simulink library "turbine_ul"  (R2018b)
settings: Solver=VariableStepAuto  StartTime=0.0  StopTime=10.0  RelTol=1e-3
libraries: vrlib x1, vectorNormalizer_ul x1
settings Model: Creator=mcobb  LastModifiedBy=mcobb

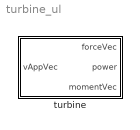
== system turbine_ul ==
  turbine : Subsystem  mask{diam=0, Cp=0, Cd=0, rho=0, rTurb=[0 1 0]}
      mask prompts: diam "Diameter"; Cp "Power Coefficient"; Cd "Drag Coefficient"; rho "Density"; rTurb "Turbine position vec"

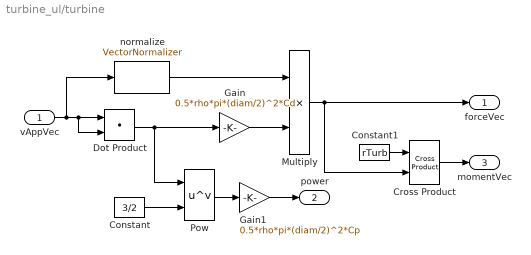
== system turbine_ul/turbine ==
  vAppVec : Inport
  Constant : Constant  Value=3/2
  Constant1 : Constant  Value=rTurb
  Cross Product : vrlib/Utilities/Cross Product
      settings: SourceProductBaseCode=VR
  Dot Product : DotProduct  InputSameDT=on  OutDataTypeStr=Inherit: Inherit via internal rule
  Gain : Gain  Gain=0.5*rho*pi*(diam/2)^2*Cd
  Gain1 : Gain  Gain=0.5*rho*pi*(diam/2)^2*Cp
  Multiply : Product
  Pow : Math  Operator=pow  RndMeth=Zero  SaturateOnIntegerOverflow=on
  "normalize " : vectorNormalizer_ul/VectorNormalizer   SystemSampleTime=-1
  forceVec : Outport
  power : Outport  Port=2
  momentVec : Outport  Port=3
  wires:
  vAppVec/1 -> "normalize "/1, Dot Product/2, Dot Product/1
  Dot Product/1 -> Pow/1, Gain/1
  Gain/1 -> Multiply/2
  "normalize "/1 -> Multiply/1
  Multiply/1 -> Cross Product/2, forceVec/1
  Gain1/1 -> power/1
  Constant/1 -> Pow/2
  Pow/1 -> Gain1/1
  Constant1/1 -> Cross Product/1
  Cross Product/1 -> momentVec/1
